simulink model "Lava_Lamp_System_For_Picture"  (R2016a)
settings: Solver=VariableStepAuto  StartTime=0.0  StopTime=10.0  RelTol=1e-3
values from neighbouring files (symbols this model uses):
  C1 = 1 / C_HEAT    (= 0.0013206550449)    [ControlDesignAndAnalysis.m]    (also in Lava_Lamp_System_Model.m)
  C2 = 1 / (R123 * C_HEAT)    (= 0.00138569660598)    [ControlDesignAndAnalysis.m]    (also in Lava_Lamp_System_Model.m)
  C3 = 1 / (R1 * C_LAVA)    (= 3.46327878577e-05)    [ControlDesignAndAnalysis.m]    (also in Lava_Lamp_System_Model.m)
  C4 = 1 / (R156 * C_LAVA)    (= 3.89625411326e-05)    [ControlDesignAndAnalysis.m]    (also in Lava_Lamp_System_Model.m)
  C5 = 1/ (R1 * C_HEAT)    (= 0.00137168160044)    [ControlDesignAndAnalysis.m]    (also in Lava_Lamp_System_Model.m)
settings Model: Creator=ddrma  LastModifiedBy=ddrma

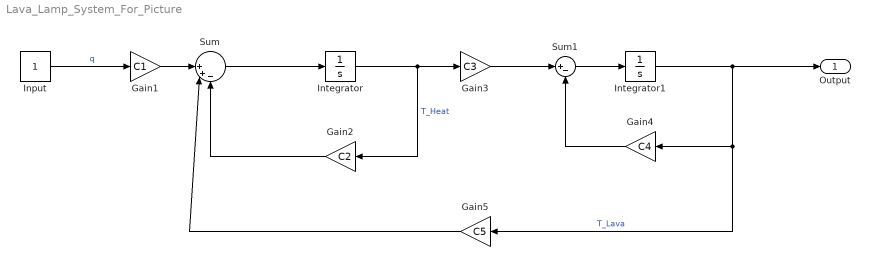
== system Lava_Lamp_System_For_Picture ==
  Gain1 : Gain  Gain=C1
  Gain2 : Gain  Gain=C2
  Gain3 : Gain  Gain=C3
  Gain4 : Gain  Gain=C4
  Gain5 : Gain  Gain=C5
  Input : Constant
  Integrator : Integrator
  Integrator1 : Integrator
  Sum : Sum  Inputs=||++-
  Sum1 : Sum  Inputs=|+-
  Output : Outport
  wires:
  Sum/1 -> Integrator/1
  Integrator/1 -> Gain2/1, Gain3/1  "T_Heat"
  Gain3/1 -> Sum1/1
  Sum1/1 -> Integrator1/1
  Gain4/1 -> Sum1/2
  Integrator1/1 -> Output/1, Gain5/1, Gain4/1  "T_Lava"
  Gain2/1 -> Sum/3
  Gain5/1 -> Sum/2
  Gain1/1 -> Sum/1
  Input/1 -> Gain1/1  "q"
